simulink model "fir6dB"  (Simulink 7.1)
settings: Solver=ode45  StartTime=0.0  StopTime=10.0  RelTol=1e-3
libraries: dsparch4 x1
settings Model: Creator=MS05572  LastModifiedBy=MS05572

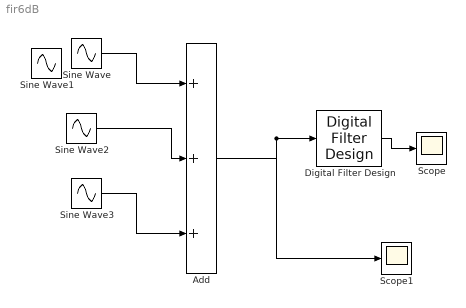
== system fir6dB ==
  Add : Sum  Inputs=+++  OutDataType=sfix(16)  OutScaling=2^-10
  Digital Filter Design : dsparch4/Digital Filter Design  SystemSampleTime=-1  mwdsp_browser_bugfix_var=off
  Scope : Scope
  Scope1 : Scope
  Sine Wave : Sin  Amplitude=5  Frequency=100*pi  SampleTime=0.001
  Sine Wave2 : Sin  Amplitude=2  Frequency=200*pi  SampleTime=0.001
  Sine Wave3 : Sin  Frequency=2*83.3*pi  SampleTime=0.001
  Sine Wave1 : Sin  IOType=siggen  SampleTime=0
  wires:
  Sine Wave/1 -> Add/1
  Sine Wave2/1 -> Add/2
  Sine Wave3/1 -> Add/3
  Add/1 -> Digital Filter Design/1, Scope1/1
  Digital Filter Design/1 -> Scope/1
